simulink model "untitled"  (R2021a)
settings: Solver=VariableStepAuto  StartTime=0.0  StopTime=5  RelTol=1e-3
settings Model: Creator=NhatDang  LastModifiedBy=NhatDang

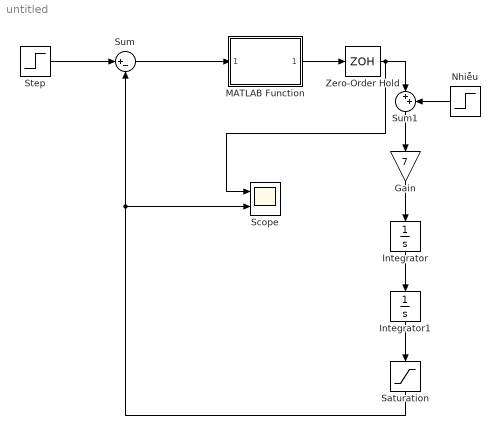
== system untitled ==
  Gain : Gain  Gain=7
  Integrator : Integrator
  Integrator1 : Integrator  InitialCondition=0.17
  MATLAB Function : MATLAB Function  TreatAsAtomicUnit=on
  Nhiễu : Step  Time=3.0  After=0.05  SampleTime=0
  Saturation : Saturate
  Scope : Scope  NumInputPorts=2
  Step : Step  Before=0.17  After=0.30  SampleTime=0
  Sum : Sum  Inputs=|+-
  Sum1 : Sum  Inputs=|++
  Zero-Order Hold : ZeroOrderHold  SampleTime=0.01
  wires:
  Step/1 -> Sum/1
  Sum/1 -> MATLAB Function/1(error_m)
  MATLAB Function/1(servo_rad) -> Zero-Order Hold/1
  Gain/1 -> Integrator/1
  Integrator/1 -> Integrator1/1
  Integrator1/1 -> Saturation/1
  Saturation/1 -> Sum/2, Scope/2
  Zero-Order Hold/1 -> Scope/1, Sum1/1
  Sum1/1 -> Gain/1
  Nhiễu/1 -> Sum1/2

== matlab function untitled/MATLAB Function ==
  settings: updateMethod=DISCRETE
  data: error_m input; servo_rad output
function servo_rad = fcn(error_m)
    % ==================================================
    % CẤU HÌNH PID
    % ==================================================
    Kp = 18.7;   
    
    Ki = 2.5;    
    
    Kd = 3.0;    
    
    % Giới hạn tích phân (Anti-Windup Limit)
    I_MAX_EFFECT = 3.0; 

    % ==================================================
    % XỬ LÝ TÍN HIỆU
    % ==================================================
    % 1. Quy đổi mét sang cm 
    error_cm = error_m * 100;
    dt = 0.01; % Sample time 10ms
    
    % 2. Khai báo biến nhớ
    persistent prev_err;
    persistent integral;
    
    if isempty(prev_err); prev_err = 0; end
    if isempty(integral); integral = 0; end
    
    % ==================================================
    % TÍNH TOÁN PID
    % ==================================================
    
    % --- P (Proportional) ---
    P_term = Kp * error_cm;
    
    % --- I (Integral) + ANTI-WINDUP ---
    % Cộng dồn lỗi
    integral = integral + (error_cm * dt);
    
    % Tính thành phần I
    I_term = Ki * integral;
    
    % [KỸ THUẬT KẸP CỔ] Anti-Windup Clamping
    % Nếu I_term quá lớn, cắt bớt ngay lập tức.
    % Giúp bi không bị vọt lố khi chạy đường dài.
    if I_term > I_MAX_EFFECT
        I_term = I_MAX_EFFECT;
        % Mẹo: Cập nhật ngược lại biến integral để nó không bị "ảo"
        integral = I_MAX_EFFECT / Ki;
    elseif I_term < -I_MAX_EFFECT
        I_term = -I_MAX_EFFECT;
        integral = -I_MAX_EFFECT / Ki;
    end
    
    % --- D (Derivative) ---
    derivative = (error_cm - prev_err) / dt;
    D_term = Kd * derivative;
    
    % --- TỔNG HỢP ---
    % Output là GÓC NGHIÊNG (Độ)
    raw_angle_deg = P_term + I_term + D_term;
    
    % ==================================================
    % GIỚI HẠN VẬT LÝ (SATURATION)
    % ==================================================
    MAX_SERVO_ANGLE = 20.0; % Góc tối đa cho phép
    
    if raw_angle_deg > MAX_SERVO_ANGLE; raw_angle_deg = MAX_SERVO_ANGLE; end
    if raw_angle_deg < -MAX_SERVO_ANGLE; raw_angle_deg = -MAX_SERVO_ANGLE; end
    
    % Đổi ra Radian trả về cho Simulink
    servo_rad = raw_angle_deg * (pi/180);
    
    % Lưu trạng thái cũ
    prev_err = error_cm;
end
